simulink model "gm_DUALportRAMinterface_v3_vnl"  (R2024a)
settings: Solver=FixedStepDiscrete  StartTime=0.0  StopTime=20  RelTol=1e-3
undefined symbols (not defined in the file or in its folder): magnitude, Ts
libraries: hdlsllib x419, hdlmdlgenlib x103, embmathops x12, simulink x5, dsphdlxfrm2 x2
(part 10 of 11)

== system gm_DUALportRAMinterface_v3_vnl/PL/integration_block1/GA_main/coefficent_array/individual1/Subsystem4 ==
  reg_in : Inport  OutDataTypeStr=fixdt(1, 33, 15)  PortDimensions=1  SampleTime=3.00000003e-08
  enable : Inport  Port=2  OutDataTypeStr=boolean  PortDimensions=1  SampleTime=3.00000003e-08
  Delay : Delay  DelayLength=1  InitialCondition=0  SampleTime=Ts
  Switch : Switch  Criteria=u2 > Threshold  OutDataTypeStr=fixdt(1, 33, 15)  SaturateOnIntegerOverflow=off  InputSameDT=off
  reg_out : Outport  SampleTime=3.00000003e-08
  wires:
  Switch/1 -> Delay/1
  enable/1 -> Switch/2
  reg_in/1 -> Switch/1
  Delay/1 -> Switch/3, reg_out/1

== system gm_DUALportRAMinterface_v3_vnl/PL/integration_block1/GA_main/coefficent_array/individual1/Subsystem5 ==
  reg_in : Inport  OutDataTypeStr=fixdt(1, 33, 15)  PortDimensions=1  SampleTime=3.00000003e-08
  enable : Inport  Port=2  OutDataTypeStr=boolean  PortDimensions=1  SampleTime=3.00000003e-08
  Delay : Delay  DelayLength=1  InitialCondition=0  SampleTime=Ts
  Switch : Switch  Criteria=u2 > Threshold  OutDataTypeStr=fixdt(1, 33, 15)  SaturateOnIntegerOverflow=off  InputSameDT=off
  reg_out : Outport  SampleTime=3.00000003e-08
  wires:
  Switch/1 -> Delay/1
  enable/1 -> Switch/2
  reg_in/1 -> Switch/1
  Delay/1 -> Switch/3, reg_out/1

== system gm_DUALportRAMinterface_v3_vnl/PL/integration_block1/GA_main/coefficent_array/individual1/Subsystem6 ==
  reg_in : Inport  OutDataTypeStr=fixdt(1, 33, 15)  PortDimensions=1  SampleTime=3.00000003e-08
  enable : Inport  Port=2  OutDataTypeStr=boolean  PortDimensions=1  SampleTime=3.00000003e-08
  Delay : Delay  DelayLength=1  InitialCondition=0  SampleTime=Ts
  Switch : Switch  Criteria=u2 > Threshold  OutDataTypeStr=fixdt(1, 33, 15)  SaturateOnIntegerOverflow=off  InputSameDT=off
  reg_out : Outport  SampleTime=3.00000003e-08
  wires:
  Switch/1 -> Delay/1
  enable/1 -> Switch/2
  reg_in/1 -> Switch/1
  Delay/1 -> Switch/3, reg_out/1

== system gm_DUALportRAMinterface_v3_vnl/PL/integration_block1/GA_main/coefficent_array/individual2/Subsystem ==
  reg_in : Inport  OutDataTypeStr=fixdt(1, 33, 15)  PortDimensions=1  SampleTime=3.00000003e-08
  enable : Inport  Port=2  OutDataTypeStr=boolean  PortDimensions=1  SampleTime=3.00000003e-08
  Delay : Delay  DelayLength=1  InitialCondition=0  SampleTime=Ts
  Switch : Switch  Criteria=u2 > Threshold  OutDataTypeStr=fixdt(1, 33, 15)  SaturateOnIntegerOverflow=off  InputSameDT=off
  reg_out : Outport  SampleTime=3.00000003e-08
  wires:
  Switch/1 -> Delay/1
  enable/1 -> Switch/2
  reg_in/1 -> Switch/1
  Delay/1 -> Switch/3, reg_out/1

== system gm_DUALportRAMinterface_v3_vnl/PL/integration_block1/GA_main/coefficent_array/individual2/Subsystem1 ==
  reg_in : Inport  OutDataTypeStr=fixdt(1, 33, 15)  PortDimensions=1  SampleTime=3.00000003e-08
  enable : Inport  Port=2  OutDataTypeStr=boolean  PortDimensions=1  SampleTime=3.00000003e-08
  Delay : Delay  DelayLength=1  InitialCondition=0  SampleTime=Ts
  Switch : Switch  Criteria=u2 > Threshold  OutDataTypeStr=fixdt(1, 33, 15)  SaturateOnIntegerOverflow=off  InputSameDT=off
  reg_out : Outport  SampleTime=3.00000003e-08
  wires:
  Switch/1 -> Delay/1
  enable/1 -> Switch/2
  reg_in/1 -> Switch/1
  Delay/1 -> Switch/3, reg_out/1

== system gm_DUALportRAMinterface_v3_vnl/PL/integration_block1/GA_main/coefficent_array/individual2/Subsystem2 ==
  reg_in : Inport  OutDataTypeStr=fixdt(1, 33, 15)  PortDimensions=1  SampleTime=3.00000003e-08
  enable : Inport  Port=2  OutDataTypeStr=boolean  PortDimensions=1  SampleTime=3.00000003e-08
  Delay : Delay  DelayLength=1  InitialCondition=0  SampleTime=Ts
  Switch : Switch  Criteria=u2 > Threshold  OutDataTypeStr=fixdt(1, 33, 15)  SaturateOnIntegerOverflow=off  InputSameDT=off
  reg_out : Outport  SampleTime=3.00000003e-08
  wires:
  Switch/1 -> Delay/1
  enable/1 -> Switch/2
  reg_in/1 -> Switch/1
  Delay/1 -> Switch/3, reg_out/1

== system gm_DUALportRAMinterface_v3_vnl/PL/integration_block1/GA_main/coefficent_array/individual2/Subsystem3 ==
  reg_in : Inport  OutDataTypeStr=fixdt(1, 33, 15)  PortDimensions=1  SampleTime=3.00000003e-08
  enable : Inport  Port=2  OutDataTypeStr=boolean  PortDimensions=1  SampleTime=3.00000003e-08
  Delay : Delay  DelayLength=1  InitialCondition=0  SampleTime=Ts
  Switch : Switch  Criteria=u2 > Threshold  OutDataTypeStr=fixdt(1, 33, 15)  SaturateOnIntegerOverflow=off  InputSameDT=off
  reg_out : Outport  SampleTime=3.00000003e-08
  wires:
  Switch/1 -> Delay/1
  enable/1 -> Switch/2
  reg_in/1 -> Switch/1
  Delay/1 -> Switch/3, reg_out/1

== system gm_DUALportRAMinterface_v3_vnl/PL/integration_block1/GA_main/coefficent_array/individual2/Subsystem4 ==
  reg_in : Inport  OutDataTypeStr=fixdt(1, 33, 15)  PortDimensions=1  SampleTime=3.00000003e-08
  enable : Inport  Port=2  OutDataTypeStr=boolean  PortDimensions=1  SampleTime=3.00000003e-08
  Delay : Delay  DelayLength=1  InitialCondition=0  SampleTime=Ts
  Switch : Switch  Criteria=u2 > Threshold  OutDataTypeStr=fixdt(1, 33, 15)  SaturateOnIntegerOverflow=off  InputSameDT=off
  reg_out : Outport  SampleTime=3.00000003e-08
  wires:
  Switch/1 -> Delay/1
  enable/1 -> Switch/2
  reg_in/1 -> Switch/1
  Delay/1 -> Switch/3, reg_out/1

== system gm_DUALportRAMinterface_v3_vnl/PL/integration_block1/GA_main/coefficent_array/individual2/Subsystem5 ==
  reg_in : Inport  OutDataTypeStr=fixdt(1, 33, 15)  PortDimensions=1  SampleTime=3.00000003e-08
  enable : Inport  Port=2  OutDataTypeStr=boolean  PortDimensions=1  SampleTime=3.00000003e-08
  Delay : Delay  DelayLength=1  InitialCondition=0  SampleTime=Ts
  Switch : Switch  Criteria=u2 > Threshold  OutDataTypeStr=fixdt(1, 33, 15)  SaturateOnIntegerOverflow=off  InputSameDT=off
  reg_out : Outport  SampleTime=3.00000003e-08
  wires:
  Switch/1 -> Delay/1
  enable/1 -> Switch/2
  reg_in/1 -> Switch/1
  Delay/1 -> Switch/3, reg_out/1

== system gm_DUALportRAMinterface_v3_vnl/PL/integration_block1/GA_main/coefficent_array/individual2/Subsystem6 ==
  reg_in : Inport  OutDataTypeStr=fixdt(1, 33, 15)  PortDimensions=1  SampleTime=3.00000003e-08
  enable : Inport  Port=2  OutDataTypeStr=boolean  PortDimensions=1  SampleTime=3.00000003e-08
  Delay : Delay  DelayLength=1  InitialCondition=0  SampleTime=Ts
  Switch : Switch  Criteria=u2 > Threshold  OutDataTypeStr=fixdt(1, 33, 15)  SaturateOnIntegerOverflow=off  InputSameDT=off
  reg_out : Outport  SampleTime=3.00000003e-08
  wires:
  Switch/1 -> Delay/1
  enable/1 -> Switch/2
  reg_in/1 -> Switch/1
  Delay/1 -> Switch/3, reg_out/1

== system gm_DUALportRAMinterface_v3_vnl/PL/integration_block1/GA_main/coefficent_array/individual3/Subsystem ==
  reg_in : Inport  OutDataTypeStr=fixdt(1, 33, 15)  PortDimensions=1  SampleTime=3.00000003e-08
  enable : Inport  Port=2  OutDataTypeStr=boolean  PortDimensions=1  SampleTime=3.00000003e-08
  Delay : Delay  DelayLength=1  InitialCondition=0  SampleTime=Ts
  Switch : Switch  Criteria=u2 > Threshold  OutDataTypeStr=fixdt(1, 33, 15)  SaturateOnIntegerOverflow=off  InputSameDT=off
  reg_out : Outport  SampleTime=3.00000003e-08
  wires:
  Switch/1 -> Delay/1
  enable/1 -> Switch/2
  reg_in/1 -> Switch/1
  Delay/1 -> Switch/3, reg_out/1

== system gm_DUALportRAMinterface_v3_vnl/PL/integration_block1/GA_main/coefficent_array/individual3/Subsystem1 ==
  reg_in : Inport  OutDataTypeStr=fixdt(1, 33, 15)  PortDimensions=1  SampleTime=3.00000003e-08
  enable : Inport  Port=2  OutDataTypeStr=boolean  PortDimensions=1  SampleTime=3.00000003e-08
  Delay : Delay  DelayLength=1  InitialCondition=0  SampleTime=Ts
  Switch : Switch  Criteria=u2 > Threshold  OutDataTypeStr=fixdt(1, 33, 15)  SaturateOnIntegerOverflow=off  InputSameDT=off
  reg_out : Outport  SampleTime=3.00000003e-08
  wires:
  Switch/1 -> Delay/1
  enable/1 -> Switch/2
  reg_in/1 -> Switch/1
  Delay/1 -> Switch/3, reg_out/1

== system gm_DUALportRAMinterface_v3_vnl/PL/integration_block1/GA_main/coefficent_array/individual3/Subsystem2 ==
  reg_in : Inport  OutDataTypeStr=fixdt(1, 33, 15)  PortDimensions=1  SampleTime=3.00000003e-08
  enable : Inport  Port=2  OutDataTypeStr=boolean  PortDimensions=1  SampleTime=3.00000003e-08
  Delay : Delay  DelayLength=1  InitialCondition=0  SampleTime=Ts
  Switch : Switch  Criteria=u2 > Threshold  OutDataTypeStr=fixdt(1, 33, 15)  SaturateOnIntegerOverflow=off  InputSameDT=off
  reg_out : Outport  SampleTime=3.00000003e-08
  wires:
  Switch/1 -> Delay/1
  enable/1 -> Switch/2
  reg_in/1 -> Switch/1
  Delay/1 -> Switch/3, reg_out/1

== system gm_DUALportRAMinterface_v3_vnl/PL/integration_block1/GA_main/coefficent_array/individual3/Subsystem3 ==
  reg_in : Inport  OutDataTypeStr=fixdt(1, 33, 15)  PortDimensions=1  SampleTime=3.00000003e-08
  enable : Inport  Port=2  OutDataTypeStr=boolean  PortDimensions=1  SampleTime=3.00000003e-08
  Delay : Delay  DelayLength=1  InitialCondition=0  SampleTime=Ts
  Switch : Switch  Criteria=u2 > Threshold  OutDataTypeStr=fixdt(1, 33, 15)  SaturateOnIntegerOverflow=off  InputSameDT=off
  reg_out : Outport  SampleTime=3.00000003e-08
  wires:
  Switch/1 -> Delay/1
  enable/1 -> Switch/2
  reg_in/1 -> Switch/1
  Delay/1 -> Switch/3, reg_out/1

== system gm_DUALportRAMinterface_v3_vnl/PL/integration_block1/GA_main/coefficent_array/individual3/Subsystem4 ==
  reg_in : Inport  OutDataTypeStr=fixdt(1, 33, 15)  PortDimensions=1  SampleTime=3.00000003e-08
  enable : Inport  Port=2  OutDataTypeStr=boolean  PortDimensions=1  SampleTime=3.00000003e-08
  Delay : Delay  DelayLength=1  InitialCondition=0  SampleTime=Ts
  Switch : Switch  Criteria=u2 > Threshold  OutDataTypeStr=fixdt(1, 33, 15)  SaturateOnIntegerOverflow=off  InputSameDT=off
  reg_out : Outport  SampleTime=3.00000003e-08
  wires:
  Switch/1 -> Delay/1
  enable/1 -> Switch/2
  reg_in/1 -> Switch/1
  Delay/1 -> Switch/3, reg_out/1

== system gm_DUALportRAMinterface_v3_vnl/PL/integration_block1/GA_main/coefficent_array/individual3/Subsystem5 ==
  reg_in : Inport  OutDataTypeStr=fixdt(1, 33, 15)  PortDimensions=1  SampleTime=3.00000003e-08
  enable : Inport  Port=2  OutDataTypeStr=boolean  PortDimensions=1  SampleTime=3.00000003e-08
  Delay : Delay  DelayLength=1  InitialCondition=0  SampleTime=Ts
  Switch : Switch  Criteria=u2 > Threshold  OutDataTypeStr=fixdt(1, 33, 15)  SaturateOnIntegerOverflow=off  InputSameDT=off
  reg_out : Outport  SampleTime=3.00000003e-08
  wires:
  Switch/1 -> Delay/1
  enable/1 -> Switch/2
  reg_in/1 -> Switch/1
  Delay/1 -> Switch/3, reg_out/1

== system gm_DUALportRAMinterface_v3_vnl/PL/integration_block1/GA_main/coefficent_array/individual3/Subsystem6 ==
  reg_in : Inport  OutDataTypeStr=fixdt(1, 33, 15)  PortDimensions=1  SampleTime=3.00000003e-08
  enable : Inport  Port=2  OutDataTypeStr=boolean  PortDimensions=1  SampleTime=3.00000003e-08
  Delay : Delay  DelayLength=1  InitialCondition=0  SampleTime=Ts
  Switch : Switch  Criteria=u2 > Threshold  OutDataTypeStr=fixdt(1, 33, 15)  SaturateOnIntegerOverflow=off  InputSameDT=off
  reg_out : Outport  SampleTime=3.00000003e-08
  wires:
  Switch/1 -> Delay/1
  enable/1 -> Switch/2
  reg_in/1 -> Switch/1
  Delay/1 -> Switch/3, reg_out/1

== system gm_DUALportRAMinterface_v3_vnl/PL/integration_block1/GA_main/coefficent_array/individual4/Subsystem ==
  reg_in : Inport  OutDataTypeStr=fixdt(1, 33, 15)  PortDimensions=1  SampleTime=3.00000003e-08
  enable : Inport  Port=2  OutDataTypeStr=boolean  PortDimensions=1  SampleTime=3.00000003e-08
  Delay : Delay  DelayLength=1  InitialCondition=0  SampleTime=Ts
  Switch : Switch  Criteria=u2 > Threshold  OutDataTypeStr=fixdt(1, 33, 15)  SaturateOnIntegerOverflow=off  InputSameDT=off
  reg_out : Outport  SampleTime=3.00000003e-08
  wires:
  Switch/1 -> Delay/1
  enable/1 -> Switch/2
  reg_in/1 -> Switch/1
  Delay/1 -> Switch/3, reg_out/1

== system gm_DUALportRAMinterface_v3_vnl/PL/integration_block1/GA_main/coefficent_array/individual4/Subsystem1 ==
  reg_in : Inport  OutDataTypeStr=fixdt(1, 33, 15)  PortDimensions=1  SampleTime=3.00000003e-08
  enable : Inport  Port=2  OutDataTypeStr=boolean  PortDimensions=1  SampleTime=3.00000003e-08
  Delay : Delay  DelayLength=1  InitialCondition=0  SampleTime=Ts
  Switch : Switch  Criteria=u2 > Threshold  OutDataTypeStr=fixdt(1, 33, 15)  SaturateOnIntegerOverflow=off  InputSameDT=off
  reg_out : Outport  SampleTime=3.00000003e-08
  wires:
  Switch/1 -> Delay/1
  enable/1 -> Switch/2
  reg_in/1 -> Switch/1
  Delay/1 -> Switch/3, reg_out/1

== system gm_DUALportRAMinterface_v3_vnl/PL/integration_block1/GA_main/coefficent_array/individual4/Subsystem2 ==
  reg_in : Inport  OutDataTypeStr=fixdt(1, 33, 15)  PortDimensions=1  SampleTime=3.00000003e-08
  enable : Inport  Port=2  OutDataTypeStr=boolean  PortDimensions=1  SampleTime=3.00000003e-08
  Delay : Delay  DelayLength=1  InitialCondition=0  SampleTime=Ts
  Switch : Switch  Criteria=u2 > Threshold  OutDataTypeStr=fixdt(1, 33, 15)  SaturateOnIntegerOverflow=off  InputSameDT=off
  reg_out : Outport  SampleTime=3.00000003e-08
  wires:
  Switch/1 -> Delay/1
  enable/1 -> Switch/2
  reg_in/1 -> Switch/1
  Delay/1 -> Switch/3, reg_out/1

== system gm_DUALportRAMinterface_v3_vnl/PL/integration_block1/GA_main/coefficent_array/individual4/Subsystem3 ==
  reg_in : Inport  OutDataTypeStr=fixdt(1, 33, 15)  PortDimensions=1  SampleTime=3.00000003e-08
  enable : Inport  Port=2  OutDataTypeStr=boolean  PortDimensions=1  SampleTime=3.00000003e-08
  Delay : Delay  DelayLength=1  InitialCondition=0  SampleTime=Ts
  Switch : Switch  Criteria=u2 > Threshold  OutDataTypeStr=fixdt(1, 33, 15)  SaturateOnIntegerOverflow=off  InputSameDT=off
  reg_out : Outport  SampleTime=3.00000003e-08
  wires:
  Switch/1 -> Delay/1
  enable/1 -> Switch/2
  reg_in/1 -> Switch/1
  Delay/1 -> Switch/3, reg_out/1

== system gm_DUALportRAMinterface_v3_vnl/PL/integration_block1/GA_main/coefficent_array/individual4/Subsystem4 ==
  reg_in : Inport  OutDataTypeStr=fixdt(1, 33, 15)  PortDimensions=1  SampleTime=3.00000003e-08
  enable : Inport  Port=2  OutDataTypeStr=boolean  PortDimensions=1  SampleTime=3.00000003e-08
  Delay : Delay  DelayLength=1  InitialCondition=0  SampleTime=Ts
  Switch : Switch  Criteria=u2 > Threshold  OutDataTypeStr=fixdt(1, 33, 15)  SaturateOnIntegerOverflow=off  InputSameDT=off
  reg_out : Outport  SampleTime=3.00000003e-08
  wires:
  Switch/1 -> Delay/1
  enable/1 -> Switch/2
  reg_in/1 -> Switch/1
  Delay/1 -> Switch/3, reg_out/1

== system gm_DUALportRAMinterface_v3_vnl/PL/integration_block1/GA_main/coefficent_array/individual4/Subsystem5 ==
  reg_in : Inport  OutDataTypeStr=fixdt(1, 33, 15)  PortDimensions=1  SampleTime=3.00000003e-08
  enable : Inport  Port=2  OutDataTypeStr=boolean  PortDimensions=1  SampleTime=3.00000003e-08
  Delay : Delay  DelayLength=1  InitialCondition=0  SampleTime=Ts
  Switch : Switch  Criteria=u2 > Threshold  OutDataTypeStr=fixdt(1, 33, 15)  SaturateOnIntegerOverflow=off  InputSameDT=off
  reg_out : Outport  SampleTime=3.00000003e-08
  wires:
  Switch/1 -> Delay/1
  enable/1 -> Switch/2
  reg_in/1 -> Switch/1
  Delay/1 -> Switch/3, reg_out/1

== system gm_DUALportRAMinterface_v3_vnl/PL/integration_block1/GA_main/coefficent_array/individual4/Subsystem6 ==
  reg_in : Inport  OutDataTypeStr=fixdt(1, 33, 15)  PortDimensions=1  SampleTime=3.00000003e-08
  enable : Inport  Port=2  OutDataTypeStr=boolean  PortDimensions=1  SampleTime=3.00000003e-08
  Delay : Delay  DelayLength=1  InitialCondition=0  SampleTime=Ts
  Switch : Switch  Criteria=u2 > Threshold  OutDataTypeStr=fixdt(1, 33, 15)  SaturateOnIntegerOverflow=off  InputSameDT=off
  reg_out : Outport  SampleTime=3.00000003e-08
  wires:
  Switch/1 -> Delay/1
  enable/1 -> Switch/2
  reg_in/1 -> Switch/1
  Delay/1 -> Switch/3, reg_out/1

== system gm_DUALportRAMinterface_v3_vnl/PL/integration_block1/GA_main/coefficent_array1/individual1/Subsystem ==
  reg_in : Inport  OutDataTypeStr=fixdt(1, 33, 15)  PortDimensions=1  SampleTime=3.00000003e-08
  enable : Inport  Port=2  OutDataTypeStr=boolean  PortDimensions=1  SampleTime=3.00000003e-08
  Delay : Delay  DelayLength=1  InitialCondition=0  SampleTime=Ts
  Switch : Switch  Criteria=u2 > Threshold  OutDataTypeStr=fixdt(1, 33, 15)  SaturateOnIntegerOverflow=off  InputSameDT=off
  reg_out : Outport  SampleTime=3.00000003e-08
  wires:
  Switch/1 -> Delay/1
  enable/1 -> Switch/2
  reg_in/1 -> Switch/1
  Delay/1 -> Switch/3, reg_out/1

== system gm_DUALportRAMinterface_v3_vnl/PL/integration_block1/GA_main/coefficent_array1/individual1/Subsystem1 ==
  reg_in : Inport  OutDataTypeStr=fixdt(1, 33, 15)  PortDimensions=1  SampleTime=3.00000003e-08
  enable : Inport  Port=2  OutDataTypeStr=boolean  PortDimensions=1  SampleTime=3.00000003e-08
  Delay : Delay  DelayLength=1  InitialCondition=0  SampleTime=Ts
  Switch : Switch  Criteria=u2 > Threshold  OutDataTypeStr=fixdt(1, 33, 15)  SaturateOnIntegerOverflow=off  InputSameDT=off
  reg_out : Outport  SampleTime=3.00000003e-08
  wires:
  Switch/1 -> Delay/1
  enable/1 -> Switch/2
  reg_in/1 -> Switch/1
  Delay/1 -> Switch/3, reg_out/1

== system gm_DUALportRAMinterface_v3_vnl/PL/integration_block1/GA_main/coefficent_array1/individual1/Subsystem2 ==
  reg_in : Inport  OutDataTypeStr=fixdt(1, 33, 15)  PortDimensions=1  SampleTime=3.00000003e-08
  enable : Inport  Port=2  OutDataTypeStr=boolean  PortDimensions=1  SampleTime=3.00000003e-08
  Delay : Delay  DelayLength=1  InitialCondition=0  SampleTime=Ts
  Switch : Switch  Criteria=u2 > Threshold  OutDataTypeStr=fixdt(1, 33, 15)  SaturateOnIntegerOverflow=off  InputSameDT=off
  reg_out : Outport  SampleTime=3.00000003e-08
  wires:
  Switch/1 -> Delay/1
  enable/1 -> Switch/2
  reg_in/1 -> Switch/1
  Delay/1 -> Switch/3, reg_out/1

== system gm_DUALportRAMinterface_v3_vnl/PL/integration_block1/GA_main/coefficent_array1/individual1/Subsystem3 ==
  reg_in : Inport  OutDataTypeStr=fixdt(1, 33, 15)  PortDimensions=1  SampleTime=3.00000003e-08
  enable : Inport  Port=2  OutDataTypeStr=boolean  PortDimensions=1  SampleTime=3.00000003e-08
  Delay : Delay  DelayLength=1  InitialCondition=0  SampleTime=Ts
  Switch : Switch  Criteria=u2 > Threshold  OutDataTypeStr=fixdt(1, 33, 15)  SaturateOnIntegerOverflow=off  InputSameDT=off
  reg_out : Outport  SampleTime=3.00000003e-08
  wires:
  Switch/1 -> Delay/1
  enable/1 -> Switch/2
  reg_in/1 -> Switch/1
  Delay/1 -> Switch/3, reg_out/1

== system gm_DUALportRAMinterface_v3_vnl/PL/integration_block1/GA_main/coefficent_array1/individual1/Subsystem4 ==
  reg_in : Inport  OutDataTypeStr=fixdt(1, 33, 15)  PortDimensions=1  SampleTime=3.00000003e-08
  enable : Inport  Port=2  OutDataTypeStr=boolean  PortDimensions=1  SampleTime=3.00000003e-08
  Delay : Delay  DelayLength=1  InitialCondition=0  SampleTime=Ts
  Switch : Switch  Criteria=u2 > Threshold  OutDataTypeStr=fixdt(1, 33, 15)  SaturateOnIntegerOverflow=off  InputSameDT=off
  reg_out : Outport  SampleTime=3.00000003e-08
  wires:
  Switch/1 -> Delay/1
  enable/1 -> Switch/2
  reg_in/1 -> Switch/1
  Delay/1 -> Switch/3, reg_out/1

== system gm_DUALportRAMinterface_v3_vnl/PL/integration_block1/GA_main/coefficent_array1/individual1/Subsystem5 ==
  reg_in : Inport  OutDataTypeStr=fixdt(1, 33, 15)  PortDimensions=1  SampleTime=3.00000003e-08
  enable : Inport  Port=2  OutDataTypeStr=boolean  PortDimensions=1  SampleTime=3.00000003e-08
  Delay : Delay  DelayLength=1  InitialCondition=0  SampleTime=Ts
  Switch : Switch  Criteria=u2 > Threshold  OutDataTypeStr=fixdt(1, 33, 15)  SaturateOnIntegerOverflow=off  InputSameDT=off
  reg_out : Outport  SampleTime=3.00000003e-08
  wires:
  Switch/1 -> Delay/1
  enable/1 -> Switch/2
  reg_in/1 -> Switch/1
  Delay/1 -> Switch/3, reg_out/1

== system gm_DUALportRAMinterface_v3_vnl/PL/integration_block1/GA_main/coefficent_array1/individual1/Subsystem6 ==
  reg_in : Inport  OutDataTypeStr=fixdt(1, 33, 15)  PortDimensions=1  SampleTime=3.00000003e-08
  enable : Inport  Port=2  OutDataTypeStr=boolean  PortDimensions=1  SampleTime=3.00000003e-08
  Delay : Delay  DelayLength=1  InitialCondition=0  SampleTime=Ts
  Switch : Switch  Criteria=u2 > Threshold  OutDataTypeStr=fixdt(1, 33, 15)  SaturateOnIntegerOverflow=off  InputSameDT=off
  reg_out : Outport  SampleTime=3.00000003e-08
  wires:
  Switch/1 -> Delay/1
  enable/1 -> Switch/2
  reg_in/1 -> Switch/1
  Delay/1 -> Switch/3, reg_out/1

== system gm_DUALportRAMinterface_v3_vnl/PL/integration_block1/GA_main/coefficent_array1/individual2/Subsystem ==
  reg_in : Inport  OutDataTypeStr=fixdt(1, 33, 15)  PortDimensions=1  SampleTime=3.00000003e-08
  enable : Inport  Port=2  OutDataTypeStr=boolean  PortDimensions=1  SampleTime=3.00000003e-08
  Delay : Delay  DelayLength=1  InitialCondition=0  SampleTime=Ts
  Switch : Switch  Criteria=u2 > Threshold  OutDataTypeStr=fixdt(1, 33, 15)  SaturateOnIntegerOverflow=off  InputSameDT=off
  reg_out : Outport  SampleTime=3.00000003e-08
  wires:
  Switch/1 -> Delay/1
  enable/1 -> Switch/2
  reg_in/1 -> Switch/1
  Delay/1 -> Switch/3, reg_out/1

== system gm_DUALportRAMinterface_v3_vnl/PL/integration_block1/GA_main/coefficent_array1/individual2/Subsystem1 ==
  reg_in : Inport  OutDataTypeStr=fixdt(1, 33, 15)  PortDimensions=1  SampleTime=3.00000003e-08
  enable : Inport  Port=2  OutDataTypeStr=boolean  PortDimensions=1  SampleTime=3.00000003e-08
  Delay : Delay  DelayLength=1  InitialCondition=0  SampleTime=Ts
  Switch : Switch  Criteria=u2 > Threshold  OutDataTypeStr=fixdt(1, 33, 15)  SaturateOnIntegerOverflow=off  InputSameDT=off
  reg_out : Outport  SampleTime=3.00000003e-08
  wires:
  Switch/1 -> Delay/1
  enable/1 -> Switch/2
  reg_in/1 -> Switch/1
  Delay/1 -> Switch/3, reg_out/1

== system gm_DUALportRAMinterface_v3_vnl/PL/integration_block1/GA_main/coefficent_array1/individual2/Subsystem2 ==
  reg_in : Inport  OutDataTypeStr=fixdt(1, 33, 15)  PortDimensions=1  SampleTime=3.00000003e-08
  enable : Inport  Port=2  OutDataTypeStr=boolean  PortDimensions=1  SampleTime=3.00000003e-08
  Delay : Delay  DelayLength=1  InitialCondition=0  SampleTime=Ts
  Switch : Switch  Criteria=u2 > Threshold  OutDataTypeStr=fixdt(1, 33, 15)  SaturateOnIntegerOverflow=off  InputSameDT=off
  reg_out : Outport  SampleTime=3.00000003e-08
  wires:
  Switch/1 -> Delay/1
  enable/1 -> Switch/2
  reg_in/1 -> Switch/1
  Delay/1 -> Switch/3, reg_out/1

== system gm_DUALportRAMinterface_v3_vnl/PL/integration_block1/GA_main/coefficent_array1/individual2/Subsystem3 ==
  reg_in : Inport  OutDataTypeStr=fixdt(1, 33, 15)  PortDimensions=1  SampleTime=3.00000003e-08
  enable : Inport  Port=2  OutDataTypeStr=boolean  PortDimensions=1  SampleTime=3.00000003e-08
  Delay : Delay  DelayLength=1  InitialCondition=0  SampleTime=Ts
  Switch : Switch  Criteria=u2 > Threshold  OutDataTypeStr=fixdt(1, 33, 15)  SaturateOnIntegerOverflow=off  InputSameDT=off
  reg_out : Outport  SampleTime=3.00000003e-08
  wires:
  Switch/1 -> Delay/1
  enable/1 -> Switch/2
  reg_in/1 -> Switch/1
  Delay/1 -> Switch/3, reg_out/1

== system gm_DUALportRAMinterface_v3_vnl/PL/integration_block1/GA_main/coefficent_array1/individual2/Subsystem4 ==
  reg_in : Inport  OutDataTypeStr=fixdt(1, 33, 15)  PortDimensions=1  SampleTime=3.00000003e-08
  enable : Inport  Port=2  OutDataTypeStr=boolean  PortDimensions=1  SampleTime=3.00000003e-08
  Delay : Delay  DelayLength=1  InitialCondition=0  SampleTime=Ts
  Switch : Switch  Criteria=u2 > Threshold  OutDataTypeStr=fixdt(1, 33, 15)  SaturateOnIntegerOverflow=off  InputSameDT=off
  reg_out : Outport  SampleTime=3.00000003e-08
  wires:
  Switch/1 -> Delay/1
  enable/1 -> Switch/2
  reg_in/1 -> Switch/1
  Delay/1 -> Switch/3, reg_out/1

== system gm_DUALportRAMinterface_v3_vnl/PL/integration_block1/GA_main/coefficent_array1/individual2/Subsystem5 ==
  reg_in : Inport  OutDataTypeStr=fixdt(1, 33, 15)  PortDimensions=1  SampleTime=3.00000003e-08
  enable : Inport  Port=2  OutDataTypeStr=boolean  PortDimensions=1  SampleTime=3.00000003e-08
  Delay : Delay  DelayLength=1  InitialCondition=0  SampleTime=Ts
  Switch : Switch  Criteria=u2 > Threshold  OutDataTypeStr=fixdt(1, 33, 15)  SaturateOnIntegerOverflow=off  InputSameDT=off
  reg_out : Outport  SampleTime=3.00000003e-08
  wires:
  Switch/1 -> Delay/1
  enable/1 -> Switch/2
  reg_in/1 -> Switch/1
  Delay/1 -> Switch/3, reg_out/1

== system gm_DUALportRAMinterface_v3_vnl/PL/integration_block1/GA_main/coefficent_array1/individual2/Subsystem6 ==
  reg_in : Inport  OutDataTypeStr=fixdt(1, 33, 15)  PortDimensions=1  SampleTime=3.00000003e-08
  enable : Inport  Port=2  OutDataTypeStr=boolean  PortDimensions=1  SampleTime=3.00000003e-08
  Delay : Delay  DelayLength=1  InitialCondition=0  SampleTime=Ts
  Switch : Switch  Criteria=u2 > Threshold  OutDataTypeStr=fixdt(1, 33, 15)  SaturateOnIntegerOverflow=off  InputSameDT=off
  reg_out : Outport  SampleTime=3.00000003e-08
  wires:
  Switch/1 -> Delay/1
  enable/1 -> Switch/2
  reg_in/1 -> Switch/1
  Delay/1 -> Switch/3, reg_out/1

== system gm_DUALportRAMinterface_v3_vnl/PL/integration_block1/GA_main/coefficent_array1/individual3/Subsystem ==
  reg_in : Inport  OutDataTypeStr=fixdt(1, 33, 15)  PortDimensions=1  SampleTime=3.00000003e-08
  enable : Inport  Port=2  OutDataTypeStr=boolean  PortDimensions=1  SampleTime=3.00000003e-08
  Delay : Delay  DelayLength=1  InitialCondition=0  SampleTime=Ts
  Switch : Switch  Criteria=u2 > Threshold  OutDataTypeStr=fixdt(1, 33, 15)  SaturateOnIntegerOverflow=off  InputSameDT=off
  reg_out : Outport  SampleTime=3.00000003e-08
  wires:
  Switch/1 -> Delay/1
  enable/1 -> Switch/2
  reg_in/1 -> Switch/1
  Delay/1 -> Switch/3, reg_out/1

== system gm_DUALportRAMinterface_v3_vnl/PL/integration_block1/GA_main/coefficent_array1/individual3/Subsystem1 ==
  reg_in : Inport  OutDataTypeStr=fixdt(1, 33, 15)  PortDimensions=1  SampleTime=3.00000003e-08
  enable : Inport  Port=2  OutDataTypeStr=boolean  PortDimensions=1  SampleTime=3.00000003e-08
  Delay : Delay  DelayLength=1  InitialCondition=0  SampleTime=Ts
  Switch : Switch  Criteria=u2 > Threshold  OutDataTypeStr=fixdt(1, 33, 15)  SaturateOnIntegerOverflow=off  InputSameDT=off
  reg_out : Outport  SampleTime=3.00000003e-08
  wires:
  Switch/1 -> Delay/1
  enable/1 -> Switch/2
  reg_in/1 -> Switch/1
  Delay/1 -> Switch/3, reg_out/1

== system gm_DUALportRAMinterface_v3_vnl/PL/integration_block1/GA_main/coefficent_array1/individual3/Subsystem2 ==
  reg_in : Inport  OutDataTypeStr=fixdt(1, 33, 15)  PortDimensions=1  SampleTime=3.00000003e-08
  enable : Inport  Port=2  OutDataTypeStr=boolean  PortDimensions=1  SampleTime=3.00000003e-08
  Delay : Delay  DelayLength=1  InitialCondition=0  SampleTime=Ts
  Switch : Switch  Criteria=u2 > Threshold  OutDataTypeStr=fixdt(1, 33, 15)  SaturateOnIntegerOverflow=off  InputSameDT=off
  reg_out : Outport  SampleTime=3.00000003e-08
  wires:
  Switch/1 -> Delay/1
  enable/1 -> Switch/2
  reg_in/1 -> Switch/1
  Delay/1 -> Switch/3, reg_out/1

== system gm_DUALportRAMinterface_v3_vnl/PL/integration_block1/GA_main/coefficent_array1/individual3/Subsystem3 ==
  reg_in : Inport  OutDataTypeStr=fixdt(1, 33, 15)  PortDimensions=1  SampleTime=3.00000003e-08
  enable : Inport  Port=2  OutDataTypeStr=boolean  PortDimensions=1  SampleTime=3.00000003e-08
  Delay : Delay  DelayLength=1  InitialCondition=0  SampleTime=Ts
  Switch : Switch  Criteria=u2 > Threshold  OutDataTypeStr=fixdt(1, 33, 15)  SaturateOnIntegerOverflow=off  InputSameDT=off
  reg_out : Outport  SampleTime=3.00000003e-08
  wires:
  Switch/1 -> Delay/1
  enable/1 -> Switch/2
  reg_in/1 -> Switch/1
  Delay/1 -> Switch/3, reg_out/1

== system gm_DUALportRAMinterface_v3_vnl/PL/integration_block1/GA_main/coefficent_array1/individual3/Subsystem4 ==
  reg_in : Inport  OutDataTypeStr=fixdt(1, 33, 15)  PortDimensions=1  SampleTime=3.00000003e-08
  enable : Inport  Port=2  OutDataTypeStr=boolean  PortDimensions=1  SampleTime=3.00000003e-08
  Delay : Delay  DelayLength=1  InitialCondition=0  SampleTime=Ts
  Switch : Switch  Criteria=u2 > Threshold  OutDataTypeStr=fixdt(1, 33, 15)  SaturateOnIntegerOverflow=off  InputSameDT=off
  reg_out : Outport  SampleTime=3.00000003e-08
  wires:
  Switch/1 -> Delay/1
  enable/1 -> Switch/2
  reg_in/1 -> Switch/1
  Delay/1 -> Switch/3, reg_out/1

== system gm_DUALportRAMinterface_v3_vnl/PL/integration_block1/GA_main/coefficent_array1/individual3/Subsystem5 ==
  reg_in : Inport  OutDataTypeStr=fixdt(1, 33, 15)  PortDimensions=1  SampleTime=3.00000003e-08
  enable : Inport  Port=2  OutDataTypeStr=boolean  PortDimensions=1  SampleTime=3.00000003e-08
  Delay : Delay  DelayLength=1  InitialCondition=0  SampleTime=Ts
  Switch : Switch  Criteria=u2 > Threshold  OutDataTypeStr=fixdt(1, 33, 15)  SaturateOnIntegerOverflow=off  InputSameDT=off
  reg_out : Outport  SampleTime=3.00000003e-08
  wires:
  Switch/1 -> Delay/1
  enable/1 -> Switch/2
  reg_in/1 -> Switch/1
  Delay/1 -> Switch/3, reg_out/1

== system gm_DUALportRAMinterface_v3_vnl/PL/integration_block1/GA_main/coefficent_array1/individual3/Subsystem6 ==
  reg_in : Inport  OutDataTypeStr=fixdt(1, 33, 15)  PortDimensions=1  SampleTime=3.00000003e-08
  enable : Inport  Port=2  OutDataTypeStr=boolean  PortDimensions=1  SampleTime=3.00000003e-08
  Delay : Delay  DelayLength=1  InitialCondition=0  SampleTime=Ts
  Switch : Switch  Criteria=u2 > Threshold  OutDataTypeStr=fixdt(1, 33, 15)  SaturateOnIntegerOverflow=off  InputSameDT=off
  reg_out : Outport  SampleTime=3.00000003e-08
  wires:
  Switch/1 -> Delay/1
  enable/1 -> Switch/2
  reg_in/1 -> Switch/1
  Delay/1 -> Switch/3, reg_out/1

== system gm_DUALportRAMinterface_v3_vnl/PL/integration_block1/GA_main/coefficent_array1/individual4/Subsystem ==
  reg_in : Inport  OutDataTypeStr=fixdt(1, 33, 15)  PortDimensions=1  SampleTime=3.00000003e-08
  enable : Inport  Port=2  OutDataTypeStr=boolean  PortDimensions=1  SampleTime=3.00000003e-08
  Delay : Delay  DelayLength=1  InitialCondition=0  SampleTime=Ts
  Switch : Switch  Criteria=u2 > Threshold  OutDataTypeStr=fixdt(1, 33, 15)  SaturateOnIntegerOverflow=off  InputSameDT=off
  reg_out : Outport  SampleTime=3.00000003e-08
  wires:
  Switch/1 -> Delay/1
  enable/1 -> Switch/2
  reg_in/1 -> Switch/1
  Delay/1 -> Switch/3, reg_out/1

== system gm_DUALportRAMinterface_v3_vnl/PL/integration_block1/GA_main/coefficent_array1/individual4/Subsystem1 ==
  reg_in : Inport  OutDataTypeStr=fixdt(1, 33, 15)  PortDimensions=1  SampleTime=3.00000003e-08
  enable : Inport  Port=2  OutDataTypeStr=boolean  PortDimensions=1  SampleTime=3.00000003e-08
  Delay : Delay  DelayLength=1  InitialCondition=0  SampleTime=Ts
  Switch : Switch  Criteria=u2 > Threshold  OutDataTypeStr=fixdt(1, 33, 15)  SaturateOnIntegerOverflow=off  InputSameDT=off
  reg_out : Outport  SampleTime=3.00000003e-08
  wires:
  Switch/1 -> Delay/1
  enable/1 -> Switch/2
  reg_in/1 -> Switch/1
  Delay/1 -> Switch/3, reg_out/1

== system gm_DUALportRAMinterface_v3_vnl/PL/integration_block1/GA_main/coefficent_array1/individual4/Subsystem2 ==
  reg_in : Inport  OutDataTypeStr=fixdt(1, 33, 15)  PortDimensions=1  SampleTime=3.00000003e-08
  enable : Inport  Port=2  OutDataTypeStr=boolean  PortDimensions=1  SampleTime=3.00000003e-08
  Delay : Delay  DelayLength=1  InitialCondition=0  SampleTime=Ts
  Switch : Switch  Criteria=u2 > Threshold  OutDataTypeStr=fixdt(1, 33, 15)  SaturateOnIntegerOverflow=off  InputSameDT=off
  reg_out : Outport  SampleTime=3.00000003e-08
  wires:
  Switch/1 -> Delay/1
  enable/1 -> Switch/2
  reg_in/1 -> Switch/1
  Delay/1 -> Switch/3, reg_out/1

== system gm_DUALportRAMinterface_v3_vnl/PL/integration_block1/GA_main/coefficent_array1/individual4/Subsystem3 ==
  reg_in : Inport  OutDataTypeStr=fixdt(1, 33, 15)  PortDimensions=1  SampleTime=3.00000003e-08
  enable : Inport  Port=2  OutDataTypeStr=boolean  PortDimensions=1  SampleTime=3.00000003e-08
  Delay : Delay  DelayLength=1  InitialCondition=0  SampleTime=Ts
  Switch : Switch  Criteria=u2 > Threshold  OutDataTypeStr=fixdt(1, 33, 15)  SaturateOnIntegerOverflow=off  InputSameDT=off
  reg_out : Outport  SampleTime=3.00000003e-08
  wires:
  Switch/1 -> Delay/1
  enable/1 -> Switch/2
  reg_in/1 -> Switch/1
  Delay/1 -> Switch/3, reg_out/1

== system gm_DUALportRAMinterface_v3_vnl/PL/integration_block1/GA_main/coefficent_array1/individual4/Subsystem4 ==
  reg_in : Inport  OutDataTypeStr=fixdt(1, 33, 15)  PortDimensions=1  SampleTime=3.00000003e-08
  enable : Inport  Port=2  OutDataTypeStr=boolean  PortDimensions=1  SampleTime=3.00000003e-08
  Delay : Delay  DelayLength=1  InitialCondition=0  SampleTime=Ts
  Switch : Switch  Criteria=u2 > Threshold  OutDataTypeStr=fixdt(1, 33, 15)  SaturateOnIntegerOverflow=off  InputSameDT=off
  reg_out : Outport  SampleTime=3.00000003e-08
  wires:
  Switch/1 -> Delay/1
  enable/1 -> Switch/2
  reg_in/1 -> Switch/1
  Delay/1 -> Switch/3, reg_out/1

== system gm_DUALportRAMinterface_v3_vnl/PL/integration_block1/GA_main/coefficent_array1/individual4/Subsystem5 ==
  reg_in : Inport  OutDataTypeStr=fixdt(1, 33, 15)  PortDimensions=1  SampleTime=3.00000003e-08
  enable : Inport  Port=2  OutDataTypeStr=boolean  PortDimensions=1  SampleTime=3.00000003e-08
  Delay : Delay  DelayLength=1  InitialCondition=0  SampleTime=Ts
  Switch : Switch  Criteria=u2 > Threshold  OutDataTypeStr=fixdt(1, 33, 15)  SaturateOnIntegerOverflow=off  InputSameDT=off
  reg_out : Outport  SampleTime=3.00000003e-08
  wires:
  Switch/1 -> Delay/1
  enable/1 -> Switch/2
  reg_in/1 -> Switch/1
  Delay/1 -> Switch/3, reg_out/1

== system gm_DUALportRAMinterface_v3_vnl/PL/integration_block1/GA_main/coefficent_array1/individual4/Subsystem6 ==
  reg_in : Inport  OutDataTypeStr=fixdt(1, 33, 15)  PortDimensions=1  SampleTime=3.00000003e-08
  enable : Inport  Port=2  OutDataTypeStr=boolean  PortDimensions=1  SampleTime=3.00000003e-08
  Delay : Delay  DelayLength=1  InitialCondition=0  SampleTime=Ts
  Switch : Switch  Criteria=u2 > Threshold  OutDataTypeStr=fixdt(1, 33, 15)  SaturateOnIntegerOverflow=off  InputSameDT=off
  reg_out : Outport  SampleTime=3.00000003e-08
  wires:
  Switch/1 -> Delay/1
  enable/1 -> Switch/2
  reg_in/1 -> Switch/1
  Delay/1 -> Switch/3, reg_out/1

== system gm_DUALportRAMinterface_v3_vnl/PL_vnl/integration_block1/GA_main/coefficent_array/individual1/Subsystem ==
  reg_in : Inport
  enable : Inport  Port=2
  Delay : Delay  DelayLength=1  InitialCondition=0  SampleTime=Ts
  Switch : Switch  Criteria=u2 > Threshold  SaturateOnIntegerOverflow=off  InputSameDT=off
  reg_out : Outport
  wires:
  reg_in/1 -> Switch/1
  enable/1 -> Switch/2
  Switch/1 -> Delay/1
  Delay/1 -> Switch/3, reg_out/1

== system gm_DUALportRAMinterface_v3_vnl/PL_vnl/integration_block1/GA_main/coefficent_array/individual1/Subsystem1 ==
  reg_in : Inport
  enable : Inport  Port=2
  Delay : Delay  DelayLength=1  InitialCondition=0  SampleTime=Ts
  Switch : Switch  Criteria=u2 > Threshold  SaturateOnIntegerOverflow=off  InputSameDT=off
  reg_out : Outport
  wires:
  reg_in/1 -> Switch/1
  enable/1 -> Switch/2
  Switch/1 -> Delay/1
  Delay/1 -> Switch/3, reg_out/1

== system gm_DUALportRAMinterface_v3_vnl/PL_vnl/integration_block1/GA_main/coefficent_array/individual1/Subsystem2 ==
  reg_in : Inport
  enable : Inport  Port=2
  Delay : Delay  DelayLength=1  InitialCondition=0  SampleTime=Ts
  Switch : Switch  Criteria=u2 > Threshold  SaturateOnIntegerOverflow=off  InputSameDT=off
  reg_out : Outport
  wires:
  reg_in/1 -> Switch/1
  enable/1 -> Switch/2
  Switch/1 -> Delay/1
  Delay/1 -> Switch/3, reg_out/1

== system gm_DUALportRAMinterface_v3_vnl/PL_vnl/integration_block1/GA_main/coefficent_array/individual1/Subsystem3 ==
  reg_in : Inport
  enable : Inport  Port=2
  Delay : Delay  DelayLength=1  InitialCondition=0  SampleTime=Ts
  Switch : Switch  Criteria=u2 > Threshold  SaturateOnIntegerOverflow=off  InputSameDT=off
  reg_out : Outport
  wires:
  reg_in/1 -> Switch/1
  enable/1 -> Switch/2
  Switch/1 -> Delay/1
  Delay/1 -> Switch/3, reg_out/1

== system gm_DUALportRAMinterface_v3_vnl/PL_vnl/integration_block1/GA_main/coefficent_array/individual1/Subsystem4 ==
  reg_in : Inport
  enable : Inport  Port=2
  Delay : Delay  DelayLength=1  InitialCondition=0  SampleTime=Ts
  Switch : Switch  Criteria=u2 > Threshold  SaturateOnIntegerOverflow=off  InputSameDT=off
  reg_out : Outport
  wires:
  reg_in/1 -> Switch/1
  enable/1 -> Switch/2
  Switch/1 -> Delay/1
  Delay/1 -> Switch/3, reg_out/1

== system gm_DUALportRAMinterface_v3_vnl/PL_vnl/integration_block1/GA_main/coefficent_array/individual1/Subsystem5 ==
  reg_in : Inport
  enable : Inport  Port=2
  Delay : Delay  DelayLength=1  InitialCondition=0  SampleTime=Ts
  Switch : Switch  Criteria=u2 > Threshold  SaturateOnIntegerOverflow=off  InputSameDT=off
  reg_out : Outport
  wires:
  reg_in/1 -> Switch/1
  enable/1 -> Switch/2
  Switch/1 -> Delay/1
  Delay/1 -> Switch/3, reg_out/1

== system gm_DUALportRAMinterface_v3_vnl/PL_vnl/integration_block1/GA_main/coefficent_array/individual1/Subsystem6 ==
  reg_in : Inport
  enable : Inport  Port=2
  Delay : Delay  DelayLength=1  InitialCondition=0  SampleTime=Ts
  Switch : Switch  Criteria=u2 > Threshold  SaturateOnIntegerOverflow=off  InputSameDT=off
  reg_out : Outport
  wires:
  Delay/1 -> reg_out/1, Switch/3
  Switch/1 -> Delay/1
  enable/1 -> Switch/2
  reg_in/1 -> Switch/1

== system gm_DUALportRAMinterface_v3_vnl/PL_vnl/integration_block1/GA_main/coefficent_array/individual2/Subsystem ==
  reg_in : Inport
  enable : Inport  Port=2
  Delay : Delay  DelayLength=1  InitialCondition=0  SampleTime=Ts
  Switch : Switch  Criteria=u2 > Threshold  SaturateOnIntegerOverflow=off  InputSameDT=off
  reg_out : Outport
  wires:
  Delay/1 -> reg_out/1, Switch/3
  Switch/1 -> Delay/1
  enable/1 -> Switch/2
  reg_in/1 -> Switch/1

== system gm_DUALportRAMinterface_v3_vnl/PL_vnl/integration_block1/GA_main/coefficent_array/individual2/Subsystem1 ==
  reg_in : Inport
  enable : Inport  Port=2
  Delay : Delay  DelayLength=1  InitialCondition=0  SampleTime=Ts
  Switch : Switch  Criteria=u2 > Threshold  SaturateOnIntegerOverflow=off  InputSameDT=off
  reg_out : Outport
  wires:
  Delay/1 -> reg_out/1, Switch/3
  Switch/1 -> Delay/1
  enable/1 -> Switch/2
  reg_in/1 -> Switch/1

== system gm_DUALportRAMinterface_v3_vnl/PL_vnl/integration_block1/GA_main/coefficent_array/individual2/Subsystem2 ==
  reg_in : Inport
  enable : Inport  Port=2
  Delay : Delay  DelayLength=1  InitialCondition=0  SampleTime=Ts
  Switch : Switch  Criteria=u2 > Threshold  SaturateOnIntegerOverflow=off  InputSameDT=off
  reg_out : Outport
  wires:
  Delay/1 -> reg_out/1, Switch/3
  Switch/1 -> Delay/1
  enable/1 -> Switch/2
  reg_in/1 -> Switch/1

== system gm_DUALportRAMinterface_v3_vnl/PL_vnl/integration_block1/GA_main/coefficent_array/individual2/Subsystem3 ==
  reg_in : Inport
  enable : Inport  Port=2
  Delay : Delay  DelayLength=1  InitialCondition=0  SampleTime=Ts
  Switch : Switch  Criteria=u2 > Threshold  SaturateOnIntegerOverflow=off  InputSameDT=off
  reg_out : Outport
  wires:
  Delay/1 -> reg_out/1, Switch/3
  Switch/1 -> Delay/1
  enable/1 -> Switch/2
  reg_in/1 -> Switch/1

== system gm_DUALportRAMinterface_v3_vnl/PL_vnl/integration_block1/GA_main/coefficent_array/individual2/Subsystem4 ==
  reg_in : Inport
  enable : Inport  Port=2
  Delay : Delay  DelayLength=1  InitialCondition=0  SampleTime=Ts
  Switch : Switch  Criteria=u2 > Threshold  SaturateOnIntegerOverflow=off  InputSameDT=off
  reg_out : Outport
  wires:
  Delay/1 -> reg_out/1, Switch/3
  Switch/1 -> Delay/1
  enable/1 -> Switch/2
  reg_in/1 -> Switch/1

== system gm_DUALportRAMinterface_v3_vnl/PL_vnl/integration_block1/GA_main/coefficent_array/individual2/Subsystem5 ==
  reg_in : Inport
  enable : Inport  Port=2
  Delay : Delay  DelayLength=1  InitialCondition=0  SampleTime=Ts
  Switch : Switch  Criteria=u2 > Threshold  SaturateOnIntegerOverflow=off  InputSameDT=off
  reg_out : Outport
  wires:
  Delay/1 -> reg_out/1, Switch/3
  Switch/1 -> Delay/1
  enable/1 -> Switch/2
  reg_in/1 -> Switch/1

== system gm_DUALportRAMinterface_v3_vnl/PL_vnl/integration_block1/GA_main/coefficent_array/individual2/Subsystem6 ==
  reg_in : Inport
  enable : Inport  Port=2
  Delay : Delay  DelayLength=1  InitialCondition=0  SampleTime=Ts
  Switch : Switch  Criteria=u2 > Threshold  SaturateOnIntegerOverflow=off  InputSameDT=off
  reg_out : Outport
  wires:
  reg_in/1 -> Switch/1
  enable/1 -> Switch/2
  Switch/1 -> Delay/1
  Delay/1 -> Switch/3, reg_out/1

== system gm_DUALportRAMinterface_v3_vnl/PL_vnl/integration_block1/GA_main/coefficent_array/individual3/Subsystem ==
  reg_in : Inport
  enable : Inport  Port=2
  Delay : Delay  DelayLength=1  InitialCondition=0  SampleTime=Ts
  Switch : Switch  Criteria=u2 > Threshold  SaturateOnIntegerOverflow=off  InputSameDT=off
  reg_out : Outport
  wires:
  reg_in/1 -> Switch/1
  enable/1 -> Switch/2
  Switch/1 -> Delay/1
  Delay/1 -> Switch/3, reg_out/1

== system gm_DUALportRAMinterface_v3_vnl/PL_vnl/integration_block1/GA_main/coefficent_array/individual3/Subsystem1 ==
  reg_in : Inport
  enable : Inport  Port=2
  Delay : Delay  DelayLength=1  InitialCondition=0  SampleTime=Ts
  Switch : Switch  Criteria=u2 > Threshold  SaturateOnIntegerOverflow=off  InputSameDT=off
  reg_out : Outport
  wires:
  reg_in/1 -> Switch/1
  enable/1 -> Switch/2
  Switch/1 -> Delay/1
  Delay/1 -> Switch/3, reg_out/1

== system gm_DUALportRAMinterface_v3_vnl/PL_vnl/integration_block1/GA_main/coefficent_array/individual3/Subsystem2 ==
  reg_in : Inport
  enable : Inport  Port=2
  Delay : Delay  DelayLength=1  InitialCondition=0  SampleTime=Ts
  Switch : Switch  Criteria=u2 > Threshold  SaturateOnIntegerOverflow=off  InputSameDT=off
  reg_out : Outport
  wires:
  reg_in/1 -> Switch/1
  enable/1 -> Switch/2
  Switch/1 -> Delay/1
  Delay/1 -> Switch/3, reg_out/1

== system gm_DUALportRAMinterface_v3_vnl/PL_vnl/integration_block1/GA_main/coefficent_array/individual3/Subsystem3 ==
  reg_in : Inport
  enable : Inport  Port=2
  Delay : Delay  DelayLength=1  InitialCondition=0  SampleTime=Ts
  Switch : Switch  Criteria=u2 > Threshold  SaturateOnIntegerOverflow=off  InputSameDT=off
  reg_out : Outport
  wires:
  reg_in/1 -> Switch/1
  enable/1 -> Switch/2
  Switch/1 -> Delay/1
  Delay/1 -> Switch/3, reg_out/1

== system gm_DUALportRAMinterface_v3_vnl/PL_vnl/integration_block1/GA_main/coefficent_array/individual3/Subsystem4 ==
  reg_in : Inport
  enable : Inport  Port=2
  Delay : Delay  DelayLength=1  InitialCondition=0  SampleTime=Ts
  Switch : Switch  Criteria=u2 > Threshold  SaturateOnIntegerOverflow=off  InputSameDT=off
  reg_out : Outport
  wires:
  reg_in/1 -> Switch/1
  enable/1 -> Switch/2
  Switch/1 -> Delay/1
  Delay/1 -> Switch/3, reg_out/1

== system gm_DUALportRAMinterface_v3_vnl/PL_vnl/integration_block1/GA_main/coefficent_array/individual3/Subsystem5 ==
  reg_in : Inport
  enable : Inport  Port=2
  Delay : Delay  DelayLength=1  InitialCondition=0  SampleTime=Ts
  Switch : Switch  Criteria=u2 > Threshold  SaturateOnIntegerOverflow=off  InputSameDT=off
  reg_out : Outport
  wires:
  reg_in/1 -> Switch/1
  enable/1 -> Switch/2
  Switch/1 -> Delay/1
  Delay/1 -> Switch/3, reg_out/1

== system gm_DUALportRAMinterface_v3_vnl/PL_vnl/integration_block1/GA_main/coefficent_array/individual3/Subsystem6 ==
  reg_in : Inport
  enable : Inport  Port=2
  Delay : Delay  DelayLength=1  InitialCondition=0  SampleTime=Ts
  Switch : Switch  Criteria=u2 > Threshold  SaturateOnIntegerOverflow=off  InputSameDT=off
  reg_out : Outport
  wires:
  Delay/1 -> reg_out/1, Switch/3
  Switch/1 -> Delay/1
  enable/1 -> Switch/2
  reg_in/1 -> Switch/1

== system gm_DUALportRAMinterface_v3_vnl/PL_vnl/integration_block1/GA_main/coefficent_array/individual4/Subsystem ==
  reg_in : Inport
  enable : Inport  Port=2
  Delay : Delay  DelayLength=1  InitialCondition=0  SampleTime=Ts
  Switch : Switch  Criteria=u2 > Threshold  SaturateOnIntegerOverflow=off  InputSameDT=off
  reg_out : Outport
  wires:
  Delay/1 -> reg_out/1, Switch/3
  Switch/1 -> Delay/1
  enable/1 -> Switch/2
  reg_in/1 -> Switch/1

== system gm_DUALportRAMinterface_v3_vnl/PL_vnl/integration_block1/GA_main/coefficent_array/individual4/Subsystem1 ==
  reg_in : Inport
  enable : Inport  Port=2
  Delay : Delay  DelayLength=1  InitialCondition=0  SampleTime=Ts
  Switch : Switch  Criteria=u2 > Threshold  SaturateOnIntegerOverflow=off  InputSameDT=off
  reg_out : Outport
  wires:
  Delay/1 -> reg_out/1, Switch/3
  Switch/1 -> Delay/1
  enable/1 -> Switch/2
  reg_in/1 -> Switch/1

== system gm_DUALportRAMinterface_v3_vnl/PL_vnl/integration_block1/GA_main/coefficent_array/individual4/Subsystem2 ==
  reg_in : Inport
  enable : Inport  Port=2
  Delay : Delay  DelayLength=1  InitialCondition=0  SampleTime=Ts
  Switch : Switch  Criteria=u2 > Threshold  SaturateOnIntegerOverflow=off  InputSameDT=off
  reg_out : Outport
  wires:
  Delay/1 -> reg_out/1, Switch/3
  Switch/1 -> Delay/1
  enable/1 -> Switch/2
  reg_in/1 -> Switch/1

== system gm_DUALportRAMinterface_v3_vnl/PL_vnl/integration_block1/GA_main/coefficent_array/individual4/Subsystem3 ==
  reg_in : Inport
  enable : Inport  Port=2
  Delay : Delay  DelayLength=1  InitialCondition=0  SampleTime=Ts
  Switch : Switch  Criteria=u2 > Threshold  SaturateOnIntegerOverflow=off  InputSameDT=off
  reg_out : Outport
  wires:
  Delay/1 -> reg_out/1, Switch/3
  Switch/1 -> Delay/1
  enable/1 -> Switch/2
  reg_in/1 -> Switch/1

== system gm_DUALportRAMinterface_v3_vnl/PL_vnl/integration_block1/GA_main/coefficent_array/individual4/Subsystem4 ==
  reg_in : Inport
  enable : Inport  Port=2
  Delay : Delay  DelayLength=1  InitialCondition=0  SampleTime=Ts
  Switch : Switch  Criteria=u2 > Threshold  SaturateOnIntegerOverflow=off  InputSameDT=off
  reg_out : Outport
  wires:
  Delay/1 -> reg_out/1, Switch/3
  Switch/1 -> Delay/1
  enable/1 -> Switch/2
  reg_in/1 -> Switch/1

== system gm_DUALportRAMinterface_v3_vnl/PL_vnl/integration_block1/GA_main/coefficent_array/individual4/Subsystem5 ==
  reg_in : Inport
  enable : Inport  Port=2
  Delay : Delay  DelayLength=1  InitialCondition=0  SampleTime=Ts
  Switch : Switch  Criteria=u2 > Threshold  SaturateOnIntegerOverflow=off  InputSameDT=off
  reg_out : Outport
  wires:
  Delay/1 -> reg_out/1, Switch/3
  Switch/1 -> Delay/1
  enable/1 -> Switch/2
  reg_in/1 -> Switch/1

== system gm_DUALportRAMinterface_v3_vnl/PL_vnl/integration_block1/GA_main/coefficent_array/individual4/Subsystem6 ==
  reg_in : Inport
  enable : Inport  Port=2
  Delay : Delay  DelayLength=1  InitialCondition=0  SampleTime=Ts
  Switch : Switch  Criteria=u2 > Threshold  SaturateOnIntegerOverflow=off  InputSameDT=off
  reg_out : Outport
  wires:
  reg_in/1 -> Switch/1
  enable/1 -> Switch/2
  Switch/1 -> Delay/1
  Delay/1 -> Switch/3, reg_out/1

== system gm_DUALportRAMinterface_v3_vnl/PL_vnl/integration_block1/GA_main/coefficent_array1/individual1/Subsystem ==
  reg_in : Inport
  enable : Inport  Port=2
  Delay : Delay  DelayLength=1  InitialCondition=0  SampleTime=Ts
  Switch : Switch  Criteria=u2 > Threshold  SaturateOnIntegerOverflow=off  InputSameDT=off
  reg_out : Outport
  wires:
  Delay/1 -> reg_out/1, Switch/3
  Switch/1 -> Delay/1
  enable/1 -> Switch/2
  reg_in/1 -> Switch/1

== system gm_DUALportRAMinterface_v3_vnl/PL_vnl/integration_block1/GA_main/coefficent_array1/individual1/Subsystem1 ==
  reg_in : Inport
  enable : Inport  Port=2
  Delay : Delay  DelayLength=1  InitialCondition=0  SampleTime=Ts
  Switch : Switch  Criteria=u2 > Threshold  SaturateOnIntegerOverflow=off  InputSameDT=off
  reg_out : Outport
  wires:
  Delay/1 -> reg_out/1, Switch/3
  Switch/1 -> Delay/1
  enable/1 -> Switch/2
  reg_in/1 -> Switch/1

== system gm_DUALportRAMinterface_v3_vnl/PL_vnl/integration_block1/GA_main/coefficent_array1/individual1/Subsystem2 ==
  reg_in : Inport
  enable : Inport  Port=2
  Delay : Delay  DelayLength=1  InitialCondition=0  SampleTime=Ts
  Switch : Switch  Criteria=u2 > Threshold  SaturateOnIntegerOverflow=off  InputSameDT=off
  reg_out : Outport
  wires:
  Delay/1 -> reg_out/1, Switch/3
  Switch/1 -> Delay/1
  enable/1 -> Switch/2
  reg_in/1 -> Switch/1

== system gm_DUALportRAMinterface_v3_vnl/PL_vnl/integration_block1/GA_main/coefficent_array1/individual1/Subsystem3 ==
  reg_in : Inport
  enable : Inport  Port=2
  Delay : Delay  DelayLength=1  InitialCondition=0  SampleTime=Ts
  Switch : Switch  Criteria=u2 > Threshold  SaturateOnIntegerOverflow=off  InputSameDT=off
  reg_out : Outport
  wires:
  Delay/1 -> reg_out/1, Switch/3
  Switch/1 -> Delay/1
  enable/1 -> Switch/2
  reg_in/1 -> Switch/1

== system gm_DUALportRAMinterface_v3_vnl/PL_vnl/integration_block1/GA_main/coefficent_array1/individual1/Subsystem4 ==
  reg_in : Inport
  enable : Inport  Port=2
  Delay : Delay  DelayLength=1  InitialCondition=0  SampleTime=Ts
  Switch : Switch  Criteria=u2 > Threshold  SaturateOnIntegerOverflow=off  InputSameDT=off
  reg_out : Outport
  wires:
  Delay/1 -> reg_out/1, Switch/3
  Switch/1 -> Delay/1
  enable/1 -> Switch/2
  reg_in/1 -> Switch/1

== system gm_DUALportRAMinterface_v3_vnl/PL_vnl/integration_block1/GA_main/coefficent_array1/individual1/Subsystem5 ==
  reg_in : Inport
  enable : Inport  Port=2
  Delay : Delay  DelayLength=1  InitialCondition=0  SampleTime=Ts
  Switch : Switch  Criteria=u2 > Threshold  SaturateOnIntegerOverflow=off  InputSameDT=off
  reg_out : Outport
  wires:
  Delay/1 -> reg_out/1, Switch/3
  Switch/1 -> Delay/1
  enable/1 -> Switch/2
  reg_in/1 -> Switch/1
